simulink library "MBDS_Subsystems"  (R2018b)
settings: Solver=ode45  StartTime=0.0  StopTime=10.0  RelTol=1e-3
undefined symbols (not defined in the file or in its folder): nbo_False, nbo_True
libraries: KIBES_Signal x1438, MBDS_Modules x44, simulink x2
(part 2 of 15)

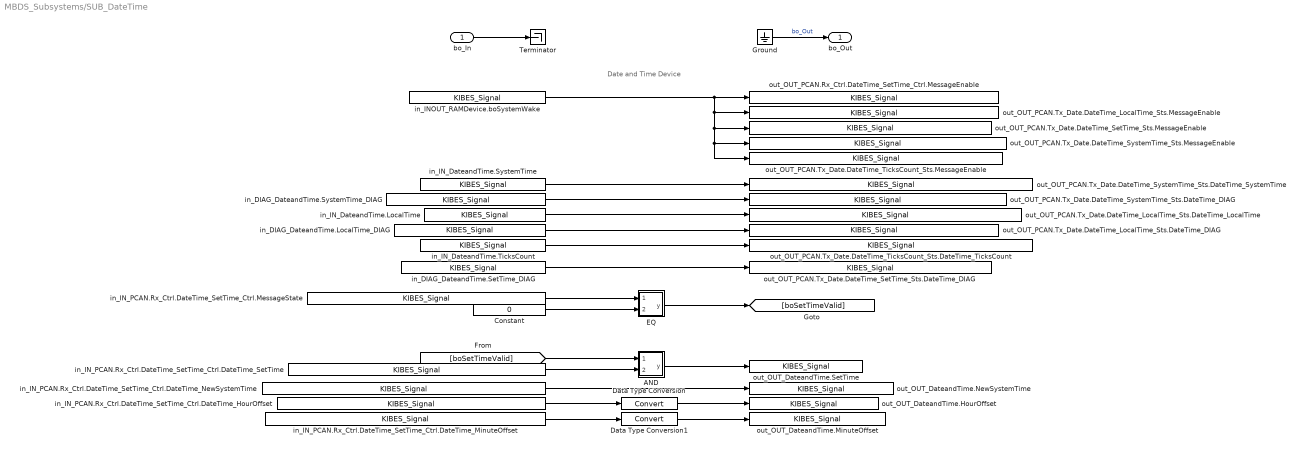
== system MBDS_Subsystems/SUB_DateTime ==
  note: Date and Time Device
  bo_In : Inport  OutDataTypeStr=boolean
  AND : Subsystem  InitFcn=|  mask(AND){MBDS_LibraryBlock=on, BitwiseMode=off, Inputs=2, UseBitMask=off, BitMask='A7', OutDataTypeStr=Inherit: Inherit via back propagation, MBDS_BlockVersion=08.20.02}
      | if(exist('MBDS_BlockCallback', 'file'))
      |    MBDS_BlockCallback('Update', gcb);
      | end
      mask prompts: MBDS_LibraryBlock "MBDS library block"; BitwiseMode "Use 'bitwise' mode"; Inputs "Number of input ports:"; UseBitMask "Use bit mask"; BitMask "Bit mask:"; OutDataTypeStr "Output data type:"; MBDS_BlockVersion "Version:"
      mask help: Logical or bitwise AND operator. For multiple inputs, operators are applied across the inputs. For a single input, operators are applied across the input vector. In bitwise mode a bit mask can be applied onto single input signals.
      mask init:
      | if(exist('MBDS_BlockCallback', 'file'))
      |    MBDS_BlockCallback('Init', gcb);
      | else
      |    % Disable all mask parameters
      |    MaskEnables = get_param(gcb, 'MaskEnables');
      |    for k = [1:length(MaskEnables)]
      |       MaskEnables{k} = 'off';
      |    end
      |    if(~isequal(MaskEnables, get_param(gcb, 'MaskEnables')))
      |       set_param(gcb, 'MaskEnables', MaskEnables);
      |    end
      | end
      mask Help: eval(['open([workdir(''library_dir:''),''\Blockset\help\'',get_param(gcb,''MaskType''),''.html''])'])
      mask Callback BitwiseMode:
      | if(exist('MBDS_BlockCallback', 'file'))
      |    MBDS_BlockCallback('BitwiseMode', gcb);
      | end
      mask Callback Inputs:
      | if(exist('MBDS_BlockCallback', 'file'))
      |    MBDS_BlockCallback('Inputs', gcb);
      | end
      mask Callback UseBitMask:
      | if(exist('MBDS_BlockCallback', 'file'))
      |    MBDS_BlockCallback('UseBitMask', gcb);
      | end
      mask Callback BitMask:
      | if(exist('MBDS_BlockCallback', 'file'))
      |    MBDS_BlockCallback('BitMask', gcb);
      | end
      mask TypeOptions OutDataTypeStr: Inherit: Inherit via back propagation | int8 | uint8 | int16 | uint16 | int32 | uint32 | boolean
      mask Callback OutDataTypeStr:
      | % Adopt Value
      | if(exist('MBDS_BlockCallback', 'file'))
      |    MBDS_BlockCallback('OutDataTypeStr', gcb);
      | end
      mask DialogControl ParameterTabVar0 Prompt: Main
      mask DialogControl ParameterTabVar01 Prompt: Signal Attributes
      mask DialogControl ParameterTabVar012 Prompt: Version
      mask Display:
      | % Show icon or block text
      | if(UseBitMask)
      |    if(isnumeric(BitMask))
      |       BitMaskString = ['0x',dec2hex(floor(BitMask))];
      |    elseif(ischar(BitMask))
      |       BitMaskString = ['0x',upper(BitMask)];
      |    else
      |       BitMaskString = '???';
      |    end
      |    disp(sprintf(['AND\n', BitMaskString]))
      | else
      |    disp('AND')
      | end
  Constant : Constant  InitFcn=|  Value=0  OutDataTypeStr=uint16
      | if(exist('MBDS_BlockCallback', 'file'))
      |    MBDS_BlockCallback('Update', gcb);  
      | end
  Data Type Conversion : DataTypeConversion  InitFcn=|
      | try
      |    MBDS_BlockCallback('Update', gcb);
      | end
      settings: AttributesFormatString=Saturate: %<SaturateOnIntegerOverflow>
  Data Type Conversion1 : DataTypeConversion  InitFcn=|
      | try
      |    MBDS_BlockCallback('Update', gcb);
      | end
      settings: AttributesFormatString=Saturate: %<SaturateOnIntegerOverflow>
  EQ : Subsystem  InitFcn=|  mask(EQ){MBDS_LibraryBlock=on, InputSameDT=on, MBDS_BlockVersion=08.20.02}
      | if(exist('MBDS_BlockCallback', 'file'))
      |    MBDS_BlockCallback('Update', gcb);
      | end
      mask prompts: MBDS_LibraryBlock "MBDS library block"; InputSameDT "Require all inputs to have the same data type"; MBDS_BlockVersion "Block version:"
      mask help: The block compares if both input signals are equal.
      mask init: same as MBDS_Subsystems/SUB_DateTime/AND
      mask Help: eval(['open([workdir(''library_dir:''),''\Blockset\help\'',get_param(gcb,''MaskType''),''.html''])'])
      mask Callback InputSameDT:
      | % Adopt value
      | if(exist('MBDS_BlockCallback', 'file'))
      |    MBDS_BlockCallback('InputSameDT', gcb);
      | end
      mask DialogControl ParameterTabVar0 Prompt: Signal Attributes
      mask DialogControl ParameterTabVar01 Prompt: Version
      mask Display:
      | % Show icon or block text
      | if(exist('MBDS_BlockCallback', 'file'))
      |    image(imread('EQ.tif','tif'),[0.35,0.35,0.355,0.25])
      |    disp('')
      | else
      |    disp(sprintf('=='));
      | end
  Ground : Ground  InitFcn=|
      | try
      |    MBDS_BlockCallback('Update', gcb);
      | end
      settings: MoveFcn=UpdateBlockSize(gcb);
  Terminator : Terminator
      settings: MoveFcn=UpdateBlockSize(gcb);
      settings: InitFcn=|
      | try
      |    MBDS_BlockCallback('Update', gcb);
      | end
  in_DIAG_DateandTime.LocalTime_DIAG : KIBES_Signal/KIBES_Signal  MBDS_LibraryBlock=on  DatabaseKey=1318  SignalName=DIAG_DateandTime.LocalTime_DIAG  SymbolName=DIAG_DateandTime_LocalTime_DIAG_001318  DataType=uint16  Init=1  Slope=1  Bias=0  DataSize=1  fpDataType=uint16  BlockIOType=Inport  DeviceType=0
  in_DIAG_DateandTime.SetTime_DIAG : KIBES_Signal/KIBES_Signal  MBDS_LibraryBlock=on  DatabaseKey=1322  SignalName=DIAG_DateandTime.SetTime_DIAG  SymbolName=DIAG_DateandTime_SetTime_DIAG_001322  DataType=uint16  Init=1  Slope=1  Bias=0  DataSize=1  fpDataType=uint16  BlockIOType=Inport  DeviceType=0
  in_DIAG_DateandTime.SystemTime_DIAG : KIBES_Signal/KIBES_Signal  MBDS_LibraryBlock=on  DatabaseKey=1324  SignalName=DIAG_DateandTime.SystemTime_DIAG  SymbolName=DIAG_DateandTime_SystemTime_DIAG_001324  DataType=uint16  Init=1  Slope=1  Bias=0  DataSize=1  fpDataType=uint16  BlockIOType=Inport  DeviceType=0
  in_INOUT_RAMDevice.boSystemWake : KIBES_Signal/KIBES_Signal  MBDS_LibraryBlock=on  DatabaseKey=3  SignalName=INOUT_RAMDevice.boSystemWake  SymbolName=INOUT_RAMDevice_boSystemWake_000003  DataType=boolean  Init=0  Slope=1  Bias=0  DataSize=1  fpDataType=boolean  BlockIOType=Inport  DeviceType=0
  in_IN_DateandTime.LocalTime : KIBES_Signal/KIBES_Signal  MBDS_LibraryBlock=on  DatabaseKey=1317  SignalName=IN_DateandTime.LocalTime  SymbolName=IN_DateandTime_LocalTime_001317  DataType=uint32  Init=0  Slope=1  Bias=0  DataSize=1  fpDataType=uint32  BlockIOType=Inport  DeviceType=0
  in_IN_DateandTime.SystemTime : KIBES_Signal/KIBES_Signal  MBDS_LibraryBlock=on  DatabaseKey=1323  SignalName=IN_DateandTime.SystemTime  SymbolName=IN_DateandTime_SystemTime_001323  DataType=uint32  Init=0  Slope=1  Bias=0  DataSize=1  fpDataType=uint32  BlockIOType=Inport  DeviceType=0
  in_IN_DateandTime.TicksCount : KIBES_Signal/KIBES_Signal  MBDS_LibraryBlock=on  DatabaseKey=1325  SignalName=IN_DateandTime.TicksCount  SymbolName=IN_DateandTime_TicksCount_001325  DataType=uint32  Init=0  Slope=1  Bias=0  DataSize=1  fpDataType=uint32  BlockIOType=Inport  DeviceType=0
  in_IN_PCAN.Rx_Ctrl.DateTime_SetTime_Ctrl.DateTime_HourOffset : KIBES_Signal/KIBES_Signal  MBDS_LibraryBlock=on  DatabaseKey=1681  SignalName=IN_PCAN.Rx_Ctrl.DateTime_SetTime_Ctrl.DateTime_HourOffset  SymbolName=IN_PCAN_Rx_Ctrl_DateTime_SetTime_Ctrl_DateTime_HourOffs_001681  DataType=uint8  Init=0  Slope=1  Bias=0  DataSize=1  fpDataType=uint8  BlockIOType=Inport  DeviceType=0
  in_IN_PCAN.Rx_Ctrl.DateTime_SetTime_Ctrl.DateTime_MinuteOffset : KIBES_Signal/KIBES_Signal  MBDS_LibraryBlock=on  DatabaseKey=1680  SignalName=IN_PCAN.Rx_Ctrl.DateTime_SetTime_Ctrl.DateTime_MinuteOffset  SymbolName=IN_PCAN_Rx_Ctrl_DateTime_SetTime_Ctrl_DateTime_MinuteOf_001680  DataType=uint8  Init=0  Slope=1  Bias=0  DataSize=1  fpDataType=uint8  BlockIOType=Inport  DeviceType=0
  in_IN_PCAN.Rx_Ctrl.DateTime_SetTime_Ctrl.DateTime_NewSystemTime : KIBES_Signal/KIBES_Signal  MBDS_LibraryBlock=on  DatabaseKey=1679  SignalName=IN_PCAN.Rx_Ctrl.DateTime_SetTime_Ctrl.DateTime_NewSystemTime  SymbolName=IN_PCAN_Rx_Ctrl_DateTime_SetTime_Ctrl_DateTime_NewSyste_001679  DataType=uint32  Init=0  Slope=1  Bias=0  DataSize=1  fpDataType=uint32  BlockIOType=Inport  DeviceType=0
  in_IN_PCAN.Rx_Ctrl.DateTime_SetTime_Ctrl.DateTime_SetTime : KIBES_Signal/KIBES_Signal  MBDS_LibraryBlock=on  DatabaseKey=1678  SignalName=IN_PCAN.Rx_Ctrl.DateTime_SetTime_Ctrl.DateTime_SetTime  SymbolName=IN_PCAN_Rx_Ctrl_DateTime_SetTime_Ctrl_DateTime_SetTime_001678  DataType=boolean  Init=0  Slope=1  Bias=0  DataSize=1  fpDataType=boolean  BlockIOType=Inport  DeviceType=0
  in_IN_PCAN.Rx_Ctrl.DateTime_SetTime_Ctrl.MessageState : KIBES_Signal/KIBES_Signal  MBDS_LibraryBlock=on  DatabaseKey=1713  SignalName=IN_PCAN.Rx_Ctrl.DateTime_SetTime_Ctrl.MessageState  SymbolName=IN_PCAN_Rx_Ctrl_DateTime_SetTime_Ctrl_MessageState_001713  DataType=uint16  Init=0  Slope=1  Bias=0  DataSize=1  fpDataType=uint16  BlockIOType=Inport  DeviceType=0
  out_OUT_DateandTime.HourOffset : KIBES_Signal/KIBES_Signal  MBDS_LibraryBlock=on  DatabaseKey=1316  SignalName=OUT_DateandTime.HourOffset  SymbolName=OUT_DateandTime_HourOffset_001316  DataType=int8  Init=0  Slope=1  Bias=0  DataSize=1  fpDataType=int8  BlockIOType=Outport  DeviceType=0
  out_OUT_DateandTime.MinuteOffset : KIBES_Signal/KIBES_Signal  MBDS_LibraryBlock=on  DatabaseKey=1319  SignalName=OUT_DateandTime.MinuteOffset  SymbolName=OUT_DateandTime_MinuteOffset_001319  DataType=int8  Init=0  Slope=1  Bias=0  DataSize=1  fpDataType=int8  BlockIOType=Outport  DeviceType=0
  out_OUT_DateandTime.NewSystemTime : KIBES_Signal/KIBES_Signal  MBDS_LibraryBlock=on  DatabaseKey=1320  SignalName=OUT_DateandTime.NewSystemTime  SymbolName=OUT_DateandTime_NewSystemTime_001320  DataType=uint32  Init=0  Slope=1  Bias=0  DataSize=1  fpDataType=uint32  BlockIOType=Outport  DeviceType=0
  out_OUT_DateandTime.SetTime : KIBES_Signal/KIBES_Signal  MBDS_LibraryBlock=on  DatabaseKey=1321  SignalName=OUT_DateandTime.SetTime  SymbolName=OUT_DateandTime_SetTime_001321  DataType=boolean  Init=0  Slope=1  Bias=0  DataSize=1  fpDataType=boolean  BlockIOType=Outport  DeviceType=0
  out_OUT_PCAN.Rx_Ctrl.DateTime_SetTime_Ctrl.MessageEnable : KIBES_Signal/KIBES_Signal  MBDS_LibraryBlock=on  DatabaseKey=1712  SignalName=OUT_PCAN.Rx_Ctrl.DateTime_SetTime_Ctrl.MessageEnable  SymbolName=OUT_PCAN_Rx_Ctrl_DateTime_SetTime_Ctrl_MessageEnable_001712  DataType=boolean  Init=0  Slope=1  Bias=0  DataSize=1  fpDataType=boolean  BlockIOType=Outport  DeviceType=0
  out_OUT_PCAN.Tx_Date.DateTime_LocalTime_Sts.DateTime_DIAG : KIBES_Signal/KIBES_Signal  MBDS_LibraryBlock=on  DatabaseKey=1806  SignalName=OUT_PCAN.Tx_Date.DateTime_LocalTime_Sts.DateTime_DIAG  SymbolName=OUT_PCAN_Tx_Date_DateTime_LocalTime_Sts_DateTime_DIAG_001806  DataType=uint16  Init=0  Slope=1  Bias=0  DataSize=1  fpDataType=uint16  BlockIOType=Outport  DeviceType=0
  out_OUT_PCAN.Tx_Date.DateTime_LocalTime_Sts.DateTime_LocalTime : KIBES_Signal/KIBES_Signal  MBDS_LibraryBlock=on  DatabaseKey=1807  SignalName=OUT_PCAN.Tx_Date.DateTime_LocalTime_Sts.DateTime_LocalTime  SymbolName=OUT_PCAN_Tx_Date_DateTime_LocalTime_Sts_DateTime_LocalT_001807  DataType=uint32  Init=0  Slope=1  Bias=0  DataSize=1  fpDataType=uint32  BlockIOType=Outport  DeviceType=0
  out_OUT_PCAN.Tx_Date.DateTime_LocalTime_Sts.MessageEnable : KIBES_Signal/KIBES_Signal  MBDS_LibraryBlock=on  DatabaseKey=1813  SignalName=OUT_PCAN.Tx_Date.DateTime_LocalTime_Sts.MessageEnable  SymbolName=OUT_PCAN_Tx_Date_DateTime_LocalTime_Sts_MessageEnable_001813  DataType=boolean  Init=0  Slope=1  Bias=0  DataSize=1  fpDataType=boolean  BlockIOType=Outport  DeviceType=0
  out_OUT_PCAN.Tx_Date.DateTime_SetTime_Sts.DateTime_DIAG : KIBES_Signal/KIBES_Signal  MBDS_LibraryBlock=on  DatabaseKey=1808  SignalName=OUT_PCAN.Tx_Date.DateTime_SetTime_Sts.DateTime_DIAG  SymbolName=OUT_PCAN_Tx_Date_DateTime_SetTime_Sts_DateTime_DIAG_001808  DataType=uint16  Init=0  Slope=1  Bias=0  DataSize=1  fpDataType=uint16  BlockIOType=Outport  DeviceType=0
  out_OUT_PCAN.Tx_Date.DateTime_SetTime_Sts.MessageEnable : KIBES_Signal/KIBES_Signal  MBDS_LibraryBlock=on  DatabaseKey=1814  SignalName=OUT_PCAN.Tx_Date.DateTime_SetTime_Sts.MessageEnable  SymbolName=OUT_PCAN_Tx_Date_DateTime_SetTime_Sts_MessageEnable_001814  DataType=boolean  Init=0  Slope=1  Bias=0  DataSize=1  fpDataType=boolean  BlockIOType=Outport  DeviceType=0
  out_OUT_PCAN.Tx_Date.DateTime_SystemTime_Sts.DateTime_DIAG : KIBES_Signal/KIBES_Signal  MBDS_LibraryBlock=on  DatabaseKey=1810  SignalName=OUT_PCAN.Tx_Date.DateTime_SystemTime_Sts.DateTime_DIAG  SymbolName=OUT_PCAN_Tx_Date_DateTime_SystemTime_Sts_DateTime_DIAG_001810  DataType=uint16  Init=0  Slope=1  Bias=0  DataSize=1  fpDataType=uint16  BlockIOType=Outport  DeviceType=0
  out_OUT_PCAN.Tx_Date.DateTime_SystemTime_Sts.DateTime_SystemTime : KIBES_Signal/KIBES_Signal  MBDS_LibraryBlock=on  DatabaseKey=1809  SignalName=OUT_PCAN.Tx_Date.DateTime_SystemTime_Sts.DateTime_SystemTime  SymbolName=OUT_PCAN_Tx_Date_DateTime_SystemTime_Sts_DateTime_Syste_001809  DataType=uint32  Init=0  Slope=1  Bias=0  DataSize=1  fpDataType=uint32  BlockIOType=Outport  DeviceType=0
  out_OUT_PCAN.Tx_Date.DateTime_SystemTime_Sts.MessageEnable : KIBES_Signal/KIBES_Signal  MBDS_LibraryBlock=on  DatabaseKey=1815  SignalName=OUT_PCAN.Tx_Date.DateTime_SystemTime_Sts.MessageEnable  SymbolName=OUT_PCAN_Tx_Date_DateTime_SystemTime_Sts_MessageEnable_001815  DataType=boolean  Init=0  Slope=1  Bias=0  DataSize=1  fpDataType=boolean  BlockIOType=Outport  DeviceType=0
  out_OUT_PCAN.Tx_Date.DateTime_TicksCount_Sts.DateTime_TicksCount : KIBES_Signal/KIBES_Signal  MBDS_LibraryBlock=on  DatabaseKey=1811  SignalName=OUT_PCAN.Tx_Date.DateTime_TicksCount_Sts.DateTime_TicksCount  SymbolName=OUT_PCAN_Tx_Date_DateTime_TicksCount_Sts_DateTime_Ticks_001811  DataType=uint32  Init=0  Slope=1  Bias=0  DataSize=1  fpDataType=uint32  BlockIOType=Outport  DeviceType=0
  out_OUT_PCAN.Tx_Date.DateTime_TicksCount_Sts.MessageEnable : KIBES_Signal/KIBES_Signal  MBDS_LibraryBlock=on  DatabaseKey=1816  SignalName=OUT_PCAN.Tx_Date.DateTime_TicksCount_Sts.MessageEnable  SymbolName=OUT_PCAN_Tx_Date_DateTime_TicksCount_Sts_MessageEnable_001816  DataType=boolean  Init=0  Slope=1  Bias=0  DataSize=1  fpDataType=boolean  BlockIOType=Outport  DeviceType=0
  bo_Out : Outport  OutDataTypeStr=boolean
  wires:
  Data Type Conversion1/1 -> out_OUT_DateandTime.MinuteOffset/1
  Data Type Conversion/1 -> out_OUT_DateandTime.HourOffset/1
  in_IN_PCAN.Rx_Ctrl.DateTime_SetTime_Ctrl.DateTime_MinuteOffset/1 -> Data Type Conversion1/1
  in_IN_PCAN.Rx_Ctrl.DateTime_SetTime_Ctrl.DateTime_HourOffset/1 -> Data Type Conversion/1
  in_IN_PCAN.Rx_Ctrl.DateTime_SetTime_Ctrl.DateTime_NewSystemTime/1 -> out_OUT_DateandTime.NewSystemTime/1
  AND/1(y) -> out_OUT_DateandTime.SetTime/1
  in_IN_PCAN.Rx_Ctrl.DateTime_SetTime_Ctrl.DateTime_SetTime/1 -> AND/2(u2)
  [boSetTimeValid] -> AND/1(u1)
  EQ/1(y) -> [boSetTimeValid]
  Constant/1 -> EQ/2(u2)
  in_IN_PCAN.Rx_Ctrl.DateTime_SetTime_Ctrl.MessageState/1 -> EQ/1(u1)
  in_DIAG_DateandTime.SetTime_DIAG/1 -> out_OUT_PCAN.Tx_Date.DateTime_SetTime_Sts.DateTime_DIAG/1
  in_IN_DateandTime.TicksCount/1 -> out_OUT_PCAN.Tx_Date.DateTime_TicksCount_Sts.DateTime_TicksCount/1
  in_DIAG_DateandTime.LocalTime_DIAG/1 -> out_OUT_PCAN.Tx_Date.DateTime_LocalTime_Sts.DateTime_DIAG/1
  in_IN_DateandTime.LocalTime/1 -> out_OUT_PCAN.Tx_Date.DateTime_LocalTime_Sts.DateTime_LocalTime/1
  in_DIAG_DateandTime.SystemTime_DIAG/1 -> out_OUT_PCAN.Tx_Date.DateTime_SystemTime_Sts.DateTime_DIAG/1
  in_IN_DateandTime.SystemTime/1 -> out_OUT_PCAN.Tx_Date.DateTime_SystemTime_Sts.DateTime_SystemTime/1
  in_INOUT_RAMDevice.boSystemWake/1 -> out_OUT_PCAN.Tx_Date.DateTime_SystemTime_Sts.MessageEnable/1, out_OUT_PCAN.Tx_Date.DateTime_TicksCount_Sts.MessageEnable/1, out_OUT_PCAN.Tx_Date.DateTime_SetTime_Sts.MessageEnable/1, out_OUT_PCAN.Tx_Date.DateTime_LocalTime_Sts.MessageEnable/1, out_OUT_PCAN.Rx_Ctrl.DateTime_SetTime_Ctrl.MessageEnable/1
  Ground/1 -> bo_Out/1  "bo_Out"
  bo_In/1 -> Terminator/1

== system MBDS_Subsystems/SUB_ExpIOControl ==
  note: Frequency Input
  note: Status
  note: Power Groups
  note: Analog Inputs
  note: Outputs
  note: Inputs
  note: Enable M-CAN Device
  note: Enable Messages
  bo_In : Inport  OutDataTypeStr=boolean
  AnalogInputs : Subsystem
  Constant : Constant  InitFcn=|  Value=true  OutDataTypeStr=boolean
      | if(exist('MBDS_BlockCallback', 'file'))
      |    MBDS_BlockCallback('Update', gcb);  
      | end
  Data Type Conversion : DataTypeConversion  InitFcn=|  SaturateOnIntegerOverflow=on
      | try
      |    MBDS_BlockCallback('Update', gcb);
      | end
      settings: AttributesFormatString=Saturate: %<SaturateOnIntegerOverflow>
  DigitalInputs : Subsystem
  FrequencyInput : Subsystem
  Ground : Ground  InitFcn=|
      | try
      |    MBDS_BlockCallback('Update', gcb);
      | end
      settings: MoveFcn=UpdateBlockSize(gcb);
  Outputs : Subsystem
  PowerGroups : Subsystem
  Terminator : Terminator
      settings: MoveFcn=UpdateBlockSize(gcb);
      settings: InitFcn=|
      | try
      |    MBDS_BlockCallback('Update', gcb);
      | end
  in_INOUT_RAMDevice.boSystemWake : KIBES_Signal/KIBES_Signal  MBDS_LibraryBlock=on  DatabaseKey=3  SignalName=INOUT_RAMDevice.boSystemWake  SymbolName=INOUT_RAMDevice_boSystemWake_000003  DataType=boolean  Init=0  Slope=1  Bias=0  DataSize=1  fpDataType=boolean  BlockIOType=Inport  DeviceType=0
  in_IN_ACAN.BSG_EXPA.IN_PWR : KIBES_Signal/KIBES_Signal  MBDS_LibraryBlock=on  DatabaseKey=838  SignalName=IN_ACAN.BSG_EXPA.IN_PWR  SymbolName=IN_ACAN_BSG_EXPA_IN_PWR_000838  DataType=uint32  Init=0  Slope=1  Bias=0  DataSize=1  fpDataType=uint32  BlockIOType=Inport  DeviceType=0
  out_OUT_FMSCAN.Tx_Exp.BSG_Expansion_Sts.BatteryVoltage : KIBES_Signal/KIBES_Signal  MBDS_LibraryBlock=on  DatabaseKey=2358  SignalName=OUT_FMSCAN.Tx_Exp.BSG_Expansion_Sts.BatteryVoltage  SymbolName=OUT_FMSCAN_Tx_Exp_BSG_Expansion_Sts_BatteryVoltage_002358  DataType=uint16  Init=0  Slope=1  Bias=0  DataSize=1  fpDataType=uint16  BlockIOType=Outport  DeviceType=0
  out_OUT_FMSCAN.Tx_Exp.BSG_Expansion_Sts.MessageEnable : KIBES_Signal/KIBES_Signal  MBDS_LibraryBlock=on  DatabaseKey=2365  SignalName=OUT_FMSCAN.Tx_Exp.BSG_Expansion_Sts.MessageEnable  SymbolName=OUT_FMSCAN_Tx_Exp_BSG_Expansion_Sts_MessageEnable_002365  DataType=boolean  Init=0  Slope=1  Bias=0  DataSize=1  fpDataType=boolean  BlockIOType=Outport  DeviceType=0
  out_OUT_MCANMaster.DeviceEnable : KIBES_Signal/KIBES_Signal  MBDS_LibraryBlock=on  DatabaseKey=800  SignalName=OUT_MCANMaster.DeviceEnable  SymbolName=OUT_MCANMaster_DeviceEnable_000800  DataType=boolean  Init=0  Slope=1  Bias=0  DataSize=1  fpDataType=boolean  BlockIOType=Outport  DeviceType=0
  bo_Out : Outport  OutDataTypeStr=boolean
  wires:
  [boSendEnable] -> FrequencyInput/1(bo_SendEnable)
  Data Type Conversion/1 -> out_OUT_FMSCAN.Tx_Exp.BSG_Expansion_Sts.BatteryVoltage/1
  in_IN_ACAN.BSG_EXPA.IN_PWR/1 -> Data Type Conversion/1
  [boSendEnable] -> out_OUT_FMSCAN.Tx_Exp.BSG_Expansion_Sts.MessageEnable/1
  [boSendEnable] -> PowerGroups/1(bo_SendEnable)
  [boSendEnable] -> AnalogInputs/1(bo_SendEnable)
  [boSendEnable] -> Outputs/1(bo_SendEnable)
  [boSendEnable] -> DigitalInputs/1(bo_SendEnable)
  Constant/1 -> out_OUT_MCANMaster.DeviceEnable/1
  in_INOUT_RAMDevice.boSystemWake/1 -> [boSendEnable]
  Ground/1 -> bo_Out/1  "bo_Out"
  bo_In/1 -> Terminator/1

== system MBDS_Subsystems/SUB_IoControl ==
  note: PMWs
  note: Analogs Supply
  note: Power Groups
  note: Analog Inputs
  note: Digital Outputs
  note: Digital Inputs
  note: Enable Output Messages
  bo_In : Inport  OutDataTypeStr=boolean
  AnalogInputs : Subsystem
  AnalogsSupply : Subsystem
  DigitalInputs : Subsystem
  DigitalOutputs : Subsystem
  Ground : Ground  InitFcn=|
      | try
      |    MBDS_BlockCallback('Update', gcb);
      | end
      settings: MoveFcn=UpdateBlockSize(gcb);
  PWMs : Subsystem
  PowerGroups : Subsystem
  Terminator : Terminator
      settings: MoveFcn=UpdateBlockSize(gcb);
      settings: InitFcn=|
      | try
      |    MBDS_BlockCallback('Update', gcb);
      | end
  in_INOUT_RAMDevice.boSystemWake : KIBES_Signal/KIBES_Signal  MBDS_LibraryBlock=on  DatabaseKey=3  SignalName=INOUT_RAMDevice.boSystemWake  SymbolName=INOUT_RAMDevice_boSystemWake_000003  DataType=boolean  Init=0  Slope=1  Bias=0  DataSize=1  fpDataType=boolean  BlockIOType=Inport  DeviceType=0
  bo_Out : Outport  OutDataTypeStr=boolean
  wires:
  [boSendEnable] -> PWMs/1(bo_SendEnable)
  [boSendEnable] -> AnalogsSupply/1(bo_SendEnable)
  [boSendEnable] -> PowerGroups/1(bo_SendEnable)
  [boSendEnable] -> AnalogInputs/1(bo_SendEnable)
  [boSendEnable] -> DigitalOutputs/1(bo_SendEnable)
  [boSendEnable] -> DigitalInputs/1(bo_SendEnable)
  in_INOUT_RAMDevice.boSystemWake/1 -> [boSendEnable]
  Ground/1 -> bo_Out/1  "bo_Out"
  bo_In/1 -> Terminator/1
